simulink model "Q3_with_controller"  (R2015b)
settings: Solver=ode1  StartTime=0.0  StopTime=20  FixedStep=0.002  MaxStep=.1  RelTol=1e-3
PreLoadFcn:
  | load_inputs
values from neighbouring files (symbols this model uses):
  r = 0.012    [Q2biv.m]    (also in Q4c.m = 0.03 * (     sin(pi*x/d)     + (1/3)*sin(3*pi*x/d)     + (1/; load_inputs.m = 0.05)
  v_P = 1    [load_inputs.m]
  w_L = v_L/r    (= 19)    [load_inputs.m]
  w_R = v_R/r    (= 21)    [load_inputs.m]
settings Model: Creator=The MathWorks, Inc.  LastModifiedBy=SooJengTan
settings DataIOCC: SaveFormat=Array
settings OptimizationCC: ExpressionDepthLimit=2147483647
settings DebuggingCC: UnderspecifiedInitializationDetection=Classic  MergeDetectMultiDrivingBlocksExec=none  SolverPrmCheckMsg=warning  FcnCallInpInsideContextMsg=UseLocalSettings  StateNameClashWarn=warning
settings HardwareCC: ProdBitPerPointer=32  ProdLargestAtomicFloat=None  ProdIntDivRoundTo=Undefined  ProdEndianess=Unspecified  ProdWordSize=32  ProdHWDeviceType=32-bit Generic
settings GRTTargetCC: GeneratePreprocessorConditionals=Disable all  CombineOutputUpdateFcns=off  GRTInterface=on
settings ConfigComp: CovModelRefEnable=Off

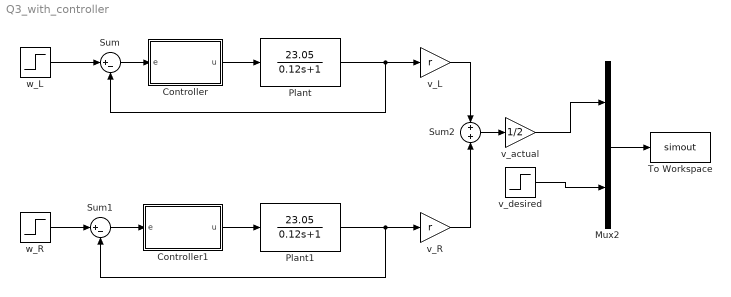
== system Q3_with_controller ==
  Controller : Subsystem
  Controller1 : Subsystem
  Mux2 : Mux  Inputs=2
  Plant : TransferFcn  Numerator=[23.05]  Denominator=[0.12 1]
  Plant1 : TransferFcn  Numerator=[23.05]  Denominator=[0.12 1]
  Sum : Sum  Inputs=|+-
  Sum1 : Sum  Inputs=|+-
  Sum2 : Sum  Inputs=+|+
  To Workspace : ToWorkspace  VariableName=simout  SaveFormat=Structure With Time  SampleTime=-1
  v_L : Gain  Gain=r
  v_R : Gain  Gain=r
  v_actual : Gain  Gain=1/2
  v_desired : Step  Time=0  After=v_P  SampleTime=0
  w_L : Step  Time=0  After=w_L  SampleTime=0
  w_R : Step  Time=0  After=w_R  SampleTime=0
  wires:
  w_L/1 -> Sum/1
  Sum/1 -> Controller/1(e)
  Plant/1 -> Sum/2, v_L/1
  w_R/1 -> Sum1/1
  Sum1/1 -> Controller1/1(e)
  Plant1/1 -> v_R/1, Sum1/2
  v_R/1 -> Sum2/2
  v_L/1 -> Sum2/1
  Sum2/1 -> v_actual/1
  Controller1/1(u) -> Plant1/1
  Controller/1(u) -> Plant/1
  v_actual/1 -> Mux2/1
  v_desired/1 -> Mux2/2
  Mux2/1 -> To Workspace/1

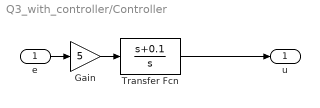
== system Q3_with_controller/Controller ==
  e : Inport
  Gain : Gain  Gain=5
  Transfer Fcn : TransferFcn  Numerator=[1 0.1]  Denominator=[1 0]
  u : Outport
  wires:
  e/1 -> Gain/1
  Transfer Fcn/1 -> u/1
  Gain/1 -> Transfer Fcn/1

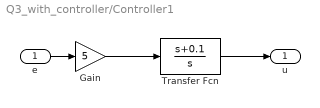
== system Q3_with_controller/Controller1 ==
  e : Inport
  Gain : Gain  Gain=5
  Transfer Fcn : TransferFcn  Numerator=[1 0.1]  Denominator=[1 0]
  u : Outport
  wires:
  e/1 -> Gain/1
  Transfer Fcn/1 -> u/1
  Gain/1 -> Transfer Fcn/1
